simulink model "Demo_1_3Q_ST250"  (Simulink 7.7)
settings: Solver=ode4  StartTime=0.0  StopTime=inf  FixedStep=sample_time_Vicon  RelTol=1e-3
InitFcn:
  | sample_time_Vicon = 0.004;
  | sample_time=0.02;
  | DeltaT = sample_time;
  | H0 = -0.36;
  | Kl = 1;
  | Omega_r =1.1; %1.3
undefined symbols (not defined in the file or in its folder): DiscIntNeverNeededParam
libraries: simulink x19, dspadpt3 x8
(part 1 of 3)
settings Model: Creator=ttcl3  LastModifiedBy=Vicon
settings SolverCC: MaxConsecutiveMinStep=auto
settings DebuggingCC: MultiTaskRateTransMsg=warning
settings SFSimCC: SimParseCustomCode=off

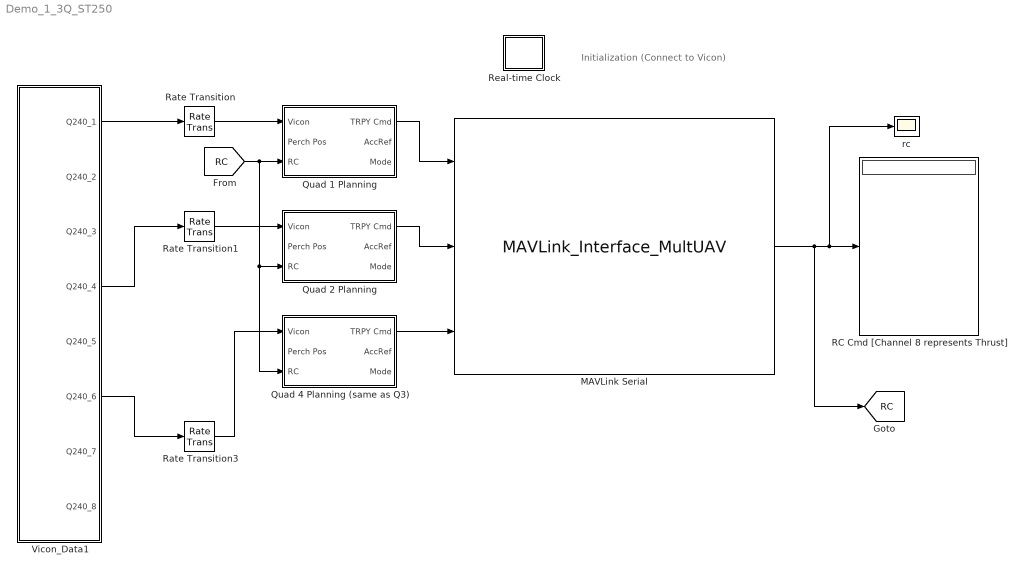
== system Demo_1_3Q_ST250 ==
  note: Initialization
      | (Connect to Vicon)
  MAVLink Serial : S-Function  FunctionName=MAVLink_Interface_MultUAV  Parameters=COM_Port,Baud_Rate,MSG_INPUT,MSG_OUTPUT  EnableBusSupport=off  mask{COM_Port='COM4', Baud_Rate=57600, RC_SCALED=on, Quad_1=on, Quad_2=on, Quad_3=on}
      mask prompts: COM_Port "COM Port"; Baud_Rate "Baud Rate"; RC_SCALED "RC CHANNELS SCALED"; Quad_1 "Quad No 1"; Quad_2 "Quad No 2"; Quad_3 "Quad No 3"
      mask init:
      | MSG_ID_NUM_INPUT = [uint8(196) uint8(197) uint8(198)];
      | MSG_ID_NAME_INPUT = [Quad_1 Quad_2 Quad_3];
      | 
      | MSG_ID_NUM_OUTPUT = [uint8(34)];
      | MSG_ID_NAME_OUTPUT = [RC_SCALED];
      | 
      | idx_input = find(MSG_ID_NAME_INPUT);
      | MSG_INPUT = MSG_ID_NUM_INPUT(idx_input);
      | 
      | idx_output = find(MSG_ID_NAME_OUTPUT);
      | MSG_OUTPUT = MSG_ID_NUM_OUTPUT(idx_output);
      mask TabNameString: Setting,Setting,Output Message,Input Message,Input Message,Input Message
      mask Display:
      | % Block image
      | image(imread('10-inch Quad Heat Map.png'));
      | 
      | %Label block
      | fprintf('MAVLink Serial\n%s\n%dbps', COM_Port,  Baud_Rate)
      | 
      | 
      | %Label input ports
      | 
      | in = 1;
      | if (Quad_1 == 1)
      |     port_label('input', in, 'Quad 1');
      |     in = in + 1;
      | end
      | if (Quad_2 == 1)
      |     port_label('input', in, 'Quad 2');
      |     in = in + 1;
      | end
      | 
      | if (Quad_3 == 1)
      |     port_label('input', in, 'Quad 3');
      |     in = in + 1;
      | end
      | 
      | %Label output ports
      | 
      | out = 1;
      | if (RC_SCALED == 1)
      |     port_label('output', out, 'RC CMD');
      |     out = out + 1;
      | end
  Quad 1 Planning : Subsystem
  Quad 2 Planning : Subsystem
  Quad 4 Planning (same as Q3) : Subsystem
  RC Cmd [Channel 8 represents Thrust] : Display
  Rate Transition : RateTransition  OutPortSampleTime=0.02
  Rate Transition1 : RateTransition  OutPortSampleTime=0.02
  Rate Transition3 : RateTransition  OutPortSampleTime=0.02
  Real-time Clock : Subsystem  mask(Real-time Clock){sample_time=sample_time, tolerance=1}
      mask prompts: sample_time "Synchronize with real-time every n seconds:"; tolerance "Real-time warning tolerance (seconds):"
      mask help: Real-time Synchronization Block
      mask Help: This block synchronizes simulation time with the PC real-time clock or UNIX system clock. The first dialog entry is the period at which the clock is checked to insure real-time synchronization. The second dialog entry is the number of seconds that the simulation time must be within real-time before a warning is printed.
      mask Display: plot(0,0,100,100,[40,60,60,54,54,64,69,76,82,77,81,83,83,81,78,74,70,64,57,49,41,35,32,30,30,31,34,40,47,47,40,40],[90,90,85,85,80,79,76,87,80,70,64,57,49,41,33,28,24,22,21,23,25,31,37,46,56,65,73,78,80,85,85,90],[69,53,53],[64,50,73])
  Vicon_Data1 : Subsystem
  rc : Scope
      settings: TimeRange=10  YMin=-1  YMax=0.1
  tag scope: RC=global
  wires:
  [RC] -> Quad 1 Planning/3(RC), Quad 2 Planning/3(RC), Quad 4 Planning (same as Q3)/3(RC)
  Quad 1 Planning/1(TRPY Cmd) -> MAVLink Serial/1
  Quad 2 Planning/1(TRPY Cmd) -> MAVLink Serial/2
  MAVLink Serial/1 -> [RC], RC Cmd [Channel 8 represents Thrust]/1, rc/1
  Rate Transition/1 -> Quad 1 Planning/1(Vicon)
  Rate Transition1/1 -> Quad 2 Planning/1(Vicon)
  Rate Transition3/1 -> Quad 4 Planning (same as Q3)/1(Vicon)
  Quad 4 Planning (same as Q3)/1(TRPY Cmd) -> MAVLink Serial/3
  Vicon_Data1/1(Q240_1) -> Rate Transition/1
  Vicon_Data1/4(Q240_4) -> Rate Transition1/1
  Vicon_Data1/6(Q240_6) -> Rate Transition3/1

== system Demo_1_3Q_ST250/Quad 1 Planning ==
  Vicon : Inport
  Perch Pos : Inport  Port=2
  RC : Inport  Port=3
  Bus Creator : BusCreator  Inputs=8
  Bus Selector : BusSelector  OutputSignals=Position,Attitude,Velocity,Acceleration
  Horizontal Pos controller : Subsystem
  Mixer : Subsystem
  Rate Transition : RateTransition  OutPortSampleTime=sample_time
  Rate Transition1 : RateTransition  OutPortSampleTime=sample_time
  Trajectory Logic : Subsystem
  Vertical Controller : Subsystem
  Yaw Controller : Subsystem
  TRPY Cmd : Outport
  AccRef : Outport  Port=2
  Mode : Outport  Port=3
  wires:
  Horizontal Pos controller/1(RPY) -> Mixer/1(RP)
  Rate Transition/1 -> Bus Creator/3  "velocity"
  Rate Transition1/1 -> Bus Creator/7  "rc"
  Bus Creator/1 -> Horizontal Pos controller/1(UAV Bus), Yaw Controller/1(UAV Bus), Vertical Controller/1(UAV bus), Trajectory Logic/1(UAV Bus)  "UAV Bus"
  Yaw Controller/1(Yaw rate des) -> Mixer/3(Yaw rate)
  Vertical Controller/1(T) -> Mixer/2(T)
  Bus Selector/4 -> Bus Creator/8  "<Acceleration>"
  Trajectory Logic/1(PosRef) -> Bus Creator/4  "position des"
  Trajectory Logic/2(attitude des) -> Bus Creator/5  "attitude des"
  Trajectory Logic/3(VelRef) -> Bus Creator/6  "velocity des"
  Trajectory Logic/5(HoverThrottle) -> Vertical Controller/2(Hover Throttle)  "Hover Throttle"
  Bus Selector/1 -> Bus Creator/1  "<Position>"
  Bus Selector/2 -> Bus Creator/2  "<Attitude>"
  Bus Selector/3 -> Rate Transition/1  "<Velocity>"
  Vicon/1 -> Bus Selector/1
  Mixer/1(XYZ RPY) -> TRPY Cmd/1
  Trajectory Logic/4(AccRef) -> AccRef/1
  Perch Pos/1 -> Trajectory Logic/2(PerchPos)
  Trajectory Logic/6(Mode) -> Mode/1
  RC/1 -> Rate Transition1/1

== system Demo_1_3Q_ST250/Quad 2 Planning ==
  Vicon : Inport
  Perch Pos : Inport  Port=2
  RC : Inport  Port=3
  Bus Creator : BusCreator  Inputs=8
  Bus Selector : BusSelector  OutputSignals=Position,Attitude,Velocity,Acceleration
  Horizontal Pos controller : Subsystem
  Mixer : Subsystem
  Rate Transition : RateTransition  OutPortSampleTime=sample_time
  Rate Transition1 : RateTransition  OutPortSampleTime=sample_time
  Trajectory Logic : Subsystem
  Vertical Controller : Subsystem
  Yaw Controller : Subsystem
  TRPY Cmd : Outport
  AccRef : Outport  Port=2
  Mode : Outport  Port=3
  wires:
  RC/1 -> Rate Transition1/1
  Trajectory Logic/6(Mode) -> Mode/1
  Perch Pos/1 -> Trajectory Logic/2(PerchPos)
  Trajectory Logic/4(AccRef) -> AccRef/1
  Mixer/1(XYZ RPY) -> TRPY Cmd/1
  Vicon/1 -> Bus Selector/1
  Bus Selector/3 -> Rate Transition/1  "<Velocity>"
  Bus Selector/2 -> Bus Creator/2  "<Attitude>"
  Bus Selector/1 -> Bus Creator/1  "<Position>"
  Trajectory Logic/5(HoverThrottle) -> Vertical Controller/2(Hover Throttle)  "Hover Throttle"
  Trajectory Logic/3(VelRef) -> Bus Creator/6  "velocity des"
  Trajectory Logic/2(attitude des) -> Bus Creator/5  "attitude des"
  Trajectory Logic/1(PosRef) -> Bus Creator/4  "position des"
  Bus Selector/4 -> Bus Creator/8  "<Acceleration>"
  Vertical Controller/1(T) -> Mixer/2(T)
  Yaw Controller/1(Yaw rate des) -> Mixer/3(Yaw rate)
  Bus Creator/1 -> Trajectory Logic/1(UAV Bus), Vertical Controller/1(UAV bus), Yaw Controller/1(UAV Bus), Horizontal Pos controller/1(UAV Bus)  "UAV Bus"
  Rate Transition1/1 -> Bus Creator/7  "rc"
  Rate Transition/1 -> Bus Creator/3  "velocity"
  Horizontal Pos controller/1(RPY) -> Mixer/1(RP)

== system Demo_1_3Q_ST250/Quad 4 Planning (same as Q3) ==
  Vicon : Inport
  Perch Pos : Inport  Port=2
  RC : Inport  Port=3
  Bus Creator : BusCreator  Inputs=8
  Bus Selector : BusSelector  OutputSignals=Position,Attitude,Velocity,Acceleration
  Horizontal Pos controller : Subsystem
  Mixer : Subsystem
  Rate Transition : RateTransition  OutPortSampleTime=sample_time
  Rate Transition1 : RateTransition  OutPortSampleTime=sample_time
  Trajectory Logic : Subsystem
  Vertical Controller : Subsystem
  Yaw Controller : Subsystem
  TRPY Cmd : Outport
  AccRef : Outport  Port=2
  Mode : Outport  Port=3
  wires:
  Horizontal Pos controller/1(RPY) -> Mixer/1(RP)
  Rate Transition/1 -> Bus Creator/3  "velocity"
  Rate Transition1/1 -> Bus Creator/7  "rc"
  Bus Creator/1 -> Horizontal Pos controller/1(UAV Bus), Yaw Controller/1(UAV Bus), Vertical Controller/1(UAV bus), Trajectory Logic/1(UAV Bus)  "UAV Bus"
  Yaw Controller/1(Yaw rate des) -> Mixer/3(Yaw rate)
  Vertical Controller/1(T) -> Mixer/2(T)
  Bus Selector/4 -> Bus Creator/8  "<Acceleration>"
  Trajectory Logic/1(PosRef) -> Bus Creator/4  "position des"
  Trajectory Logic/2(attitude des) -> Bus Creator/5  "attitude des"
  Trajectory Logic/3(VelRef) -> Bus Creator/6  "velocity des"
  Trajectory Logic/5(HoverThrottle) -> Vertical Controller/2(Hover Throttle)  "Hover Throttle"
  Bus Selector/1 -> Bus Creator/1  "<Position>"
  Bus Selector/2 -> Bus Creator/2  "<Attitude>"
  Bus Selector/3 -> Rate Transition/1  "<Velocity>"
  Vicon/1 -> Bus Selector/1
  Mixer/1(XYZ RPY) -> TRPY Cmd/1
  Trajectory Logic/4(AccRef) -> AccRef/1
  Perch Pos/1 -> Trajectory Logic/2(PerchPos)
  Trajectory Logic/6(Mode) -> Mode/1
  RC/1 -> Rate Transition1/1

== system Demo_1_3Q_ST250/Real-time Clock ==
  Real-time Clock : S-Function  FunctionName=rtclock  Parameters=sample_time, tolerance  EnableBusSupport=off

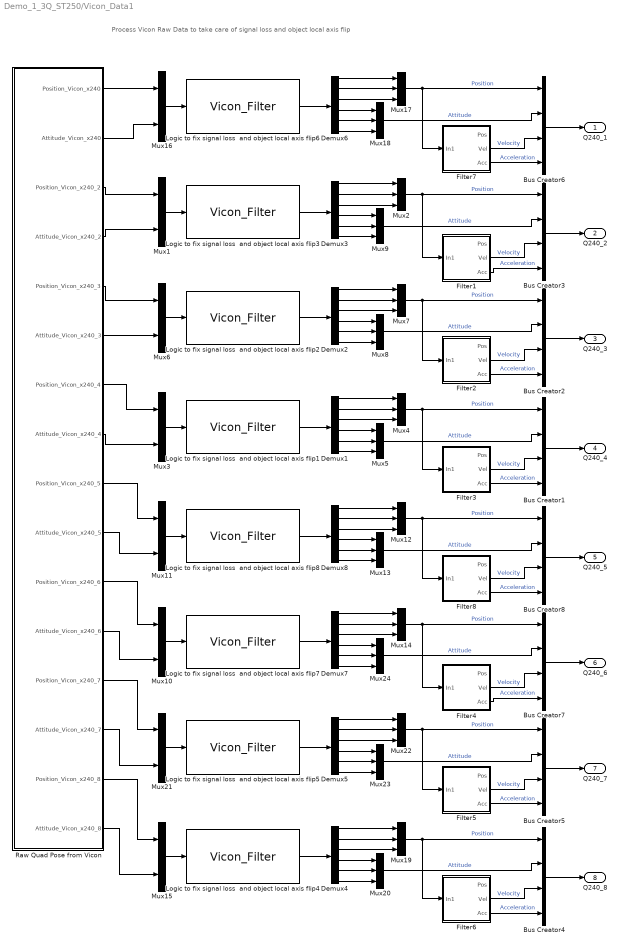
== system Demo_1_3Q_ST250/Vicon_Data1 ==
  note: Process Vicon Raw Data to take care of signal loss and object local axis flip
  Bus Creator{1..8} (8 alike) : BusCreator
  Demux{1..8} (8 alike) : Demux  Outputs=6
  Filter1 : Subsystem
  Filter2 : Subsystem
  Filter3 : Subsystem
  Filter4 : Subsystem
  Filter5 : Subsystem
  Filter6 : Subsystem
  Filter7 : Subsystem
  Filter8 : Subsystem
  Logic to fix signal loss  and object local axis flip{1..8} (8 alike) : M-S-Function  FunctionName=Vicon_Filter
  Mux{1,3,6,10..11,15..16,21} (8 alike) : Mux  Inputs=2
  Mux{2,4..5,7..9,12..14,17..20,22..24} (16 alike) : Mux  Inputs=3
  Raw Quad Pose from Vicon : Subsystem
  Q240_1 : Outport
  Q240_2 : Outport  Port=2
  Q240_3 : Outport  Port=3
  Q240_4 : Outport  Port=4
  Q240_5 : Outport  Port=5
  Q240_6 : Outport  Port=6
  Q240_7 : Outport  Port=7
  Q240_8 : Outport  Port=8
  wires:
  Mux6/1 -> Logic to fix signal loss  and object local axis flip2/1
  Logic to fix signal loss  and object local axis flip2/1 -> Demux2/1
  Demux2/1 -> Mux7/1
  Demux2/2 -> Mux7/2
  Demux2/3 -> Mux7/3
  Demux2/4 -> Mux8/1
  Demux2/5 -> Mux8/2
  Demux2/6 -> Mux8/3
  Filter2/2(Vel) -> Bus Creator2/3  "Velocity"
  Mux7/1 -> Bus Creator2/1, Filter2/1(In1)  "Position"
  Filter2/3(Acc) -> Bus Creator2/4  "Acceleration"
  Mux8/1 -> Bus Creator2/2  "Attitude"
  Bus Creator2/1 -> Q240_3/1
  Mux1/1 -> Logic to fix signal loss  and object local axis flip3/1
  Logic to fix signal loss  and object local axis flip3/1 -> Demux3/1
  Demux3/1 -> Mux2/1
  Demux3/2 -> Mux2/2
  Demux3/3 -> Mux2/3
  Demux3/4 -> Mux9/1
  Demux3/5 -> Mux9/2
  Demux3/6 -> Mux9/3
  Filter1/2(Vel) -> Bus Creator3/3  "Velocity"
  Mux2/1 -> Bus Creator3/1, Filter1/1(In1)  "Position"
  Filter1/3(Acc) -> Bus Creator3/4  "Acceleration"
  Mux9/1 -> Bus Creator3/2  "Attitude"
  Bus Creator3/1 -> Q240_2/1
  Mux16/1 -> Logic to fix signal loss  and object local axis flip6/1
  Logic to fix signal loss  and object local axis flip6/1 -> Demux6/1
  Demux6/1 -> Mux17/1
  Demux6/2 -> Mux17/2
  Demux6/3 -> Mux17/3
  Demux6/4 -> Mux18/1
  Demux6/5 -> Mux18/2
  Demux6/6 -> Mux18/3
  Filter7/2(Vel) -> Bus Creator6/3  "Velocity"
  Mux17/1 -> Bus Creator6/1, Filter7/1(In1)  "Position"
  Filter7/3(Acc) -> Bus Creator6/4  "Acceleration"
  Mux18/1 -> Bus Creator6/2  "Attitude"
  Bus Creator6/1 -> Q240_1/1
  Raw Quad Pose from Vicon/1(Position_Vicon_x240) -> Mux16/1
  Raw Quad Pose from Vicon/2(Attitude_Vicon_x240) -> Mux16/2
  Raw Quad Pose from Vicon/3(Position_Vicon_x240_2) -> Mux1/1
  Raw Quad Pose from Vicon/4(Attitude_Vicon_x240_2) -> Mux1/2
  Mux3/1 -> Logic to fix signal loss  and object local axis flip1/1
  Logic to fix signal loss  and object local axis flip1/1 -> Demux1/1
  Demux1/2 -> Mux4/2
  Demux1/3 -> Mux4/3
  Demux1/4 -> Mux5/1
  Demux1/5 -> Mux5/2
  Demux1/6 -> Mux5/3
  Filter3/2(Vel) -> Bus Creator1/3  "Velocity"
  Mux4/1 -> Filter3/1(In1), Bus Creator1/1  "Position"
  Filter3/3(Acc) -> Bus Creator1/4  "Acceleration"
  Mux5/1 -> Bus Creator1/2  "Attitude"
  Bus Creator1/1 -> Q240_4/1
  Demux1/1 -> Mux4/1
  Raw Quad Pose from Vicon/5(Position_Vicon_x240_3) -> Mux6/1
  Raw Quad Pose from Vicon/6(Attitude_Vicon_x240_3) -> Mux6/2
  Raw Quad Pose from Vicon/7(Position_Vicon_x240_4) -> Mux3/1
  Raw Quad Pose from Vicon/8(Attitude_Vicon_x240_4) -> Mux3/2
  Mux21/1 -> Logic to fix signal loss  and object local axis flip5/1
  Logic to fix signal loss  and object local axis flip5/1 -> Demux5/1
  Demux5/1 -> Mux22/1
  Demux5/2 -> Mux22/2
  Demux5/3 -> Mux22/3
  Demux5/4 -> Mux23/1
  Demux5/5 -> Mux23/2
  Demux5/6 -> Mux23/3
  Filter5/2(Vel) -> Bus Creator5/3  "Velocity"
  Mux22/1 -> Filter5/1(In1), Bus Creator5/1  "Position"
  Filter5/3(Acc) -> Bus Creator5/4  "Acceleration"
  Mux23/1 -> Bus Creator5/2  "Attitude"
  Bus Creator5/1 -> Q240_7/1
  Mux10/1 -> Logic to fix signal loss  and object local axis flip7/1
  Logic to fix signal loss  and object local axis flip7/1 -> Demux7/1
  Demux7/1 -> Mux14/1
  Demux7/2 -> Mux14/2
  Demux7/3 -> Mux14/3
  Demux7/4 -> Mux24/1
  Demux7/5 -> Mux24/2
  Demux7/6 -> Mux24/3
  Filter4/2(Vel) -> Bus Creator7/3  "Velocity"
  Mux14/1 -> Filter4/1(In1), Bus Creator7/1  "Position"
  Filter4/3(Acc) -> Bus Creator7/4  "Acceleration"
  Mux24/1 -> Bus Creator7/2  "Attitude"
  Bus Creator7/1 -> Q240_6/1
  Mux11/1 -> Logic to fix signal loss  and object local axis flip8/1
  Logic to fix signal loss  and object local axis flip8/1 -> Demux8/1
  Demux8/1 -> Mux12/1
  Demux8/2 -> Mux12/2
  Demux8/3 -> Mux12/3
  Demux8/4 -> Mux13/1
  Demux8/5 -> Mux13/2
  Demux8/6 -> Mux13/3
  Filter8/2(Vel) -> Bus Creator8/3  "Velocity"
  Mux12/1 -> Filter8/1(In1), Bus Creator8/1  "Position"
  Filter8/3(Acc) -> Bus Creator8/4  "Acceleration"
  Mux13/1 -> Bus Creator8/2  "Attitude"
  Bus Creator8/1 -> Q240_5/1
  Mux15/1 -> Logic to fix signal loss  and object local axis flip4/1
  Logic to fix signal loss  and object local axis flip4/1 -> Demux4/1
  Demux4/2 -> Mux19/2
  Demux4/3 -> Mux19/3
  Demux4/4 -> Mux20/1
  Demux4/5 -> Mux20/2
  Demux4/6 -> Mux20/3
  Filter6/2(Vel) -> Bus Creator4/3  "Velocity"
  Mux19/1 -> Bus Creator4/1, Filter6/1(In1)  "Position"
  Filter6/3(Acc) -> Bus Creator4/4  "Acceleration"
  Mux20/1 -> Bus Creator4/2  "Attitude"
  Bus Creator4/1 -> Q240_8/1
  Demux4/1 -> Mux19/1
  Raw Quad Pose from Vicon/9(Position_Vicon_x240_5) -> Mux11/1
  Raw Quad Pose from Vicon/10(Attitude_Vicon_x240_5) -> Mux11/2
  Raw Quad Pose from Vicon/11(Position_Vicon_x240_6) -> Mux10/1
  Raw Quad Pose from Vicon/12(Attitude_Vicon_x240_6) -> Mux10/2
  Raw Quad Pose from Vicon/13(Position_Vicon_x240_7) -> Mux21/1
  Raw Quad Pose from Vicon/14(Attitude_Vicon_x240_7) -> Mux21/2
  Raw Quad Pose from Vicon/15(Position_Vicon_x240_8) -> Mux15/1
  Raw Quad Pose from Vicon/16(Attitude_Vicon_x240_8) -> Mux15/2

== system Demo_1_3Q_ST250/Quad 1 Planning/Horizontal Pos controller ==
  UAV Bus : Inport
  Bus Selector : BusSelector  OutputSignals=Position,Attitude,velocity,position des,attitude des,velocity des,rc
  Horizontal Position Controller : Subsystem
  Mux1 : Mux  Inputs=2
  Mux2 : Mux  Inputs=2
  "P Ref1 " : Scope
      settings: TimeRange=10  YMin=-1.5  YMax=1.5  SaveName=ScopeData2
  Pd VS P (Q1) : Scope
      settings: TimeRange=10  YMin=-0.5  YMax=1.5  SaveName=ScopeData16
  Vd VS V : Scope
      settings: TimeRange=10  YMin=-4  YMax=4
  RPY : Outport
  wires:
  UAV Bus/1 -> Horizontal Position Controller/1(UAV Bus), Bus Selector/1
  Horizontal Position Controller/1(RPY) -> RPY/1
  Bus Selector/2 -> ?  "<Attitude>"
  Bus Selector/3 -> Mux2/1  "<velocity>"
  Bus Selector/5 -> ?  "<attitude des>"
  Bus Selector/1 -> Mux1/1, "P Ref1 "/1  "<Position>"
  Bus Selector/4 -> Mux1/2  "<position des>"
  Mux1/1 -> Pd VS P (Q1)/1
  Bus Selector/6 -> Mux2/2  "<velocity des>"
  Bus Selector/7 -> ?  "<rc>"
  Mux2/1 -> Vd VS V/1

== system Demo_1_3Q_ST250/Quad 1 Planning/Mixer ==
  note: 7x1 vector (usec, XYZRPY)
  RP : Inport
  T : Inport  Port=2
  Yaw rate : Inport  Port=3
  Mux1 : Mux  Inputs=5
  PWM : Constant  Value=0
  id : Constant
  XYZ RPY : Outport
  wires:
  Mux1/1 -> XYZ RPY/1
  T/1 -> Mux1/1
  RP/1 -> Mux1/2
  Yaw rate/1 -> Mux1/3
  PWM/1 -> Mux1/4
  id/1 -> Mux1/5

== system Demo_1_3Q_ST250/Quad 1 Planning/Trajectory Logic ==
  UAV Bus : Inport
  PerchPos : Inport  Port=2
  Bus Selector : BusSelector  OutputSignals=rc,Position,Attitude
  CommandRefSystem : Subsystem
  Mux : Mux  Inputs=2
  Selector1 : Selector  InputPortWidth=3  IndexOptions=Index vector (dialog)  Indices=[3]  OutputSizes=1
  UAV SF : Stateflow chart  TreatAsAtomicUnit=on
  PosRef : Outport
  attitude des : Outport  Port=2
  VelRef : Outport  Port=3
  AccRef : Outport  Port=4
  HoverThrottle : Outport  Port=5
  Mode : Outport  Port=6
  wires:
  UAV SF/1(PosDesired) -> CommandRefSystem/1(PosCom)
  CommandRefSystem/1(position des) -> PosRef/1
  CommandRefSystem/3(velocity des) -> VelRef/1
  Bus Selector/1 -> UAV SF/1(RC)  "<rc>"
  CommandRefSystem/4(acc des) -> AccRef/1
  UAV SF/2(HoverThrottle) -> HoverThrottle/1
  PerchPos/1 -> UAV SF/3(PerchPos)
  UAV SF/3(Mode) -> Mode/1
  UAV Bus/1 -> Bus Selector/1
  CommandRefSystem/2(attitude des) -> attitude des/1
  Bus Selector/2 -> Mux/1  "<Position>"
  Bus Selector/3 -> Selector1/1  "<Attitude>"
  Selector1/1 -> Mux/2
  Mux/1 -> UAV SF/2(Pos)

== system Demo_1_3Q_ST250/Quad 1 Planning/Vertical Controller ==
  note: Manual Thrust
  UAV bus : Inport
  Hover Throttle : Inport  Port=2
  Bus Selector : BusSelector  OutputSignals=Position,position des,rc,velocity,velocity des
  Bus Selector3 : BusSelector  OutputSignals=rc
  Selector{1,3..5} (4 alike) : Selector  InputPortWidth=3  IndexOptions=Index vector (dialog)  Indices=[3]  OutputSizes=1
  Selector2 : Selector  InputPortWidth=8  IndexOptions=Index vector (dialog)  Indices=[1]  OutputSizes=1
  Selector7 : Selector  InputPortWidth=8  IndexOptions=Index vector (dialog)  Indices=[7]  OutputSizes=1
  Sum : Sum  Inputs=|-+
  Sum1 : Sum  Inputs=|-+
  Verticall Pos Controller : Subsystem
  T : Outport
  wires:
  UAV bus/1 -> Bus Selector/1
  Bus Selector/3 -> Bus Selector3/1, Selector2/1  "<rc>"
  Bus Selector/1 -> Selector4/1  "<Position>"
  Bus Selector/2 -> Selector1/1  "<position des>"
  Sum/1 -> Verticall Pos Controller/1(Pos Error)  "Down error"
  Selector4/1 -> Sum/1
  Selector1/1 -> Sum/2
  Bus Selector3/1 -> Selector7/1  "<rc>"
  Selector7/1 -> Verticall Pos Controller/2(Reset)  "reset"
  Sum1/1 -> Verticall Pos Controller/3(Vel Error)  "Vel_error"
  Selector3/1 -> Sum1/1
  Selector5/1 -> Sum1/2
  Bus Selector/4 -> Selector3/1  "<velocity>"
  Bus Selector/5 -> Selector5/1  "<velocity des>"
  Verticall Pos Controller/1("T  Commands [-1, 1]") -> T/1  "T"
  Hover Throttle/1 -> Verticall Pos Controller/4(Hover Throttle)

== system Demo_1_3Q_ST250/Quad 1 Planning/Yaw Controller ==
  UAV Bus : Inport
  Bus Selector1 : BusSelector  OutputSignals=Attitude,attitude des,rc
  Gain : Gain  Gain=180/pi
  Heading : simulink/Continuous/PID Controller  SystemSampleTime=-1  Controller=PI  TimeDomain=Discrete-time  SampleTime=sample_time  IntegratorMethod=Trapezoidal  FilterMethod=Trapezoidal  Form=Parallel  P=2  I=1  D=0  N=100  InitialConditionSource=internal  InitialConditionForIntegrator=0  InitialConditionForFilter=0  ExternalReset=rising  LimitOutput=on  UpperSaturationLimit=300*pi/180  LowerSaturationLimit=-300*pi/180  LinearizeAsGain=off  AntiWindupMode=none  Kb=1  TrackingMode=off  Kt=1  PParamMin=[]  PParamMax=[]  IParamMin=[]  IParamMax=[]  DParamMin=[]  DParamMax=[]  NParamMin=[]  NParamMax=[]  KbParamMin=[]  KbParamMax=[]  KtParamMin=[]  KtParamMax=[]  POutMin=[]  POutMax=[]  IOutMin=[]  IOutMax=[]  DOutMin=[]  DOutMax=[]  NOutMin=[]  NOutMax=[]  KbOutMin=[]  KbOutMax=[]  KtOutMin=[]  KtOutMax=[]  IntegratorOutMin=[]  IntegratorOutMax=[]  FilterOutMin=[]  FilterOutMax=[]  SumOutMin=[]  SumOutMax=[]  SumI1OutMin=[]  SumI1OutMax=[]  SumI2OutMin=[]  SumI2OutMax=[]  SumI3OutMin=[]  SumI3OutMax=[]  SumDOutMin=[]  SumDOutMax=[]  SaturationOutMin=[]  SaturationOutMax=[]  IntegratorContinuousStateAttributes=''  IntegratorStateMustResolveToSignalObject=off  IntegratorRTWStateStorageClass=Auto  FilterContinuousStateAttributes=''  FilterStateMustResolveToSignalObject=off  FilterRTWStateStorageClass=Auto
  MATLAB Function : Stateflow chart  TreatAsAtomicUnit=on
  Selector5 : Selector  InputPortWidth=3  IndexOptions=Index vector (dialog)  Indices=[3]  OutputSizes=1
  Selector6 : Selector  InputPortWidth=3  IndexOptions=Index vector (dialog)  Indices=[3]  OutputSizes=1
  Selector7 : Selector  InputPortWidth=8  IndexOptions=Index vector (dialog)  Indices=[5]  OutputSizes=1
  Sum1 : Sum  Inputs=|-+
  Yaw rate des : Outport
  wires:
  Gain/1 -> Yaw rate des/1
  Selector5/1 -> Sum1/1
  Selector7/1 -> Heading/2  "reset"
  Heading/1 -> Gain/1  "desire yaw rate"
  Bus Selector1/1 -> Selector5/1  "<Attitude>"
  UAV Bus/1 -> Bus Selector1/1
  MATLAB Function/1(y) -> Heading/1
  Sum1/1 -> MATLAB Function/1(u)
  Selector6/1 -> Sum1/2
  Bus Selector1/2 -> Selector6/1  "<attitude des>"
  Bus Selector1/3 -> Selector7/1  "<rc>"

== system Demo_1_3Q_ST250/Quad 2 Planning/Horizontal Pos controller ==
  UAV Bus : Inport
  Bus Selector : BusSelector  OutputSignals=Position,Attitude,velocity,position des,attitude des,velocity des,rc
  Horizontal Position Controller : Subsystem
  Mux1 : Mux  Inputs=2
  Mux2 : Mux  Inputs=2
  Pd VS P (Q2) : Scope
      settings: TimeRange=10  YMin=-1.9  YMax=0  SaveName=ScopeData16
  Vd VS V : Scope
      settings: TimeRange=10  YMin=-4  YMax=4
  RPY : Outport
  wires:
  Mux2/1 -> Vd VS V/1
  Bus Selector/7 -> ?  "<rc>"
  Bus Selector/6 -> Mux2/2  "<velocity des>"
  Mux1/1 -> Pd VS P (Q2)/1
  Bus Selector/4 -> Mux1/2  "<position des>"
  Bus Selector/1 -> Mux1/1  "<Position>"
  Bus Selector/5 -> ?  "<attitude des>"
  Bus Selector/3 -> Mux2/1  "<velocity>"
  Bus Selector/2 -> ?  "<Attitude>"
  Horizontal Position Controller/1(RPY) -> RPY/1
  UAV Bus/1 -> Bus Selector/1, Horizontal Position Controller/1(UAV Bus)

== system Demo_1_3Q_ST250/Quad 2 Planning/Mixer ==
  note: 7x1 vector (usec, XYZRPY)
  RP : Inport
  T : Inport  Port=2
  Yaw rate : Inport  Port=3
  Mux1 : Mux  Inputs=5
  PWM : Constant  Value=0
  id : Constant  Value=4
  XYZ RPY : Outport
  wires:
  id/1 -> Mux1/5
  PWM/1 -> Mux1/4
  Yaw rate/1 -> Mux1/3
  RP/1 -> Mux1/2
  T/1 -> Mux1/1
  Mux1/1 -> XYZ RPY/1

== system Demo_1_3Q_ST250/Quad 2 Planning/Trajectory Logic ==
  UAV Bus : Inport
  PerchPos : Inport  Port=2
  Bus Selector : BusSelector  OutputSignals=rc,Position,Attitude
  CommandRefSystem : Subsystem
  Mux : Mux  Inputs=2
  Selector1 : Selector  InputPortWidth=3  IndexOptions=Index vector (dialog)  Indices=[3]  OutputSizes=1
  UAV SF : Stateflow chart  TreatAsAtomicUnit=on
  PosRef : Outport
  attitude des : Outport  Port=2
  VelRef : Outport  Port=3
  AccRef : Outport  Port=4
  HoverThrottle : Outport  Port=5
  Mode : Outport  Port=6
  wires:
  Mux/1 -> UAV SF/2(Pos)
  Selector1/1 -> Mux/2
  Bus Selector/3 -> Selector1/1  "<Attitude>"
  Bus Selector/2 -> Mux/1  "<Position>"
  CommandRefSystem/2(attitude des) -> attitude des/1
  UAV Bus/1 -> Bus Selector/1
  UAV SF/3(Mode) -> Mode/1
  PerchPos/1 -> UAV SF/3(PerchPos)
  UAV SF/2(HoverThrottle) -> HoverThrottle/1
  CommandRefSystem/4(acc des) -> AccRef/1
  Bus Selector/1 -> UAV SF/1(RC)  "<rc>"
  CommandRefSystem/3(velocity des) -> VelRef/1
  CommandRefSystem/1(position des) -> PosRef/1
  UAV SF/1(PosDesired) -> CommandRefSystem/1(PosCom)

== system Demo_1_3Q_ST250/Quad 2 Planning/Vertical Controller ==
  note: Manual Thrust
  UAV bus : Inport
  Hover Throttle : Inport  Port=2
  Bus Selector : BusSelector  OutputSignals=Position,position des,rc,velocity,velocity des
  Bus Selector3 : BusSelector  OutputSignals=rc
  Selector{1,3..5} (4 alike) : Selector  InputPortWidth=3  IndexOptions=Index vector (dialog)  Indices=[3]  OutputSizes=1
  Selector2 : Selector  InputPortWidth=8  IndexOptions=Index vector (dialog)  Indices=[1]  OutputSizes=1
  Selector7 : Selector  InputPortWidth=8  IndexOptions=Index vector (dialog)  Indices=[7]  OutputSizes=1
  Sum : Sum  Inputs=|-+
  Sum1 : Sum  Inputs=|-+
  Verticall Pos Controller : Subsystem
  T : Outport
  wires:
  Hover Throttle/1 -> Verticall Pos Controller/4(Hover Throttle)
  Verticall Pos Controller/1("T  Commands [-1, 1]") -> T/1  "T"
  Bus Selector/5 -> Selector5/1  "<velocity des>"
  Bus Selector/4 -> Selector3/1  "<velocity>"
  Selector5/1 -> Sum1/2
  Selector3/1 -> Sum1/1
  Sum1/1 -> Verticall Pos Controller/3(Vel Error)  "Vel_error"
  Selector7/1 -> Verticall Pos Controller/2(Reset)  "reset"
  Bus Selector3/1 -> Selector7/1  "<rc>"
  Selector1/1 -> Sum/2
  Selector4/1 -> Sum/1
  Sum/1 -> Verticall Pos Controller/1(Pos Error)  "Down error"
  Bus Selector/2 -> Selector1/1  "<position des>"
  Bus Selector/1 -> Selector4/1  "<Position>"
  Bus Selector/3 -> Selector2/1, Bus Selector3/1  "<rc>"
  UAV bus/1 -> Bus Selector/1

== system Demo_1_3Q_ST250/Quad 2 Planning/Yaw Controller ==
  UAV Bus : Inport
  Bus Selector1 : BusSelector  OutputSignals=Attitude,attitude des,rc
  Gain : Gain  Gain=180/pi
  Heading : simulink/Continuous/PID Controller  SystemSampleTime=-1  Controller=PI  TimeDomain=Discrete-time  SampleTime=sample_time  IntegratorMethod=Trapezoidal  FilterMethod=Trapezoidal  Form=Parallel  P=2  I=1  D=0  N=100  InitialConditionSource=internal  InitialConditionForIntegrator=0  InitialConditionForFilter=0  ExternalReset=rising  LimitOutput=on  UpperSaturationLimit=300*pi/180  LowerSaturationLimit=-300*pi/180  LinearizeAsGain=off  AntiWindupMode=none  Kb=1  TrackingMode=off  Kt=1  PParamMin=[]  PParamMax=[]  IParamMin=[]  IParamMax=[]  DParamMin=[]  DParamMax=[]  NParamMin=[]  NParamMax=[]  KbParamMin=[]  KbParamMax=[]  KtParamMin=[]  KtParamMax=[]  POutMin=[]  POutMax=[]  IOutMin=[]  IOutMax=[]  DOutMin=[]  DOutMax=[]  NOutMin=[]  NOutMax=[]  KbOutMin=[]  KbOutMax=[]  KtOutMin=[]  KtOutMax=[]  IntegratorOutMin=[]  IntegratorOutMax=[]  FilterOutMin=[]  FilterOutMax=[]  SumOutMin=[]  SumOutMax=[]  SumI1OutMin=[]  SumI1OutMax=[]  SumI2OutMin=[]  SumI2OutMax=[]  SumI3OutMin=[]  SumI3OutMax=[]  SumDOutMin=[]  SumDOutMax=[]  SaturationOutMin=[]  SaturationOutMax=[]  IntegratorContinuousStateAttributes=''  IntegratorStateMustResolveToSignalObject=off  IntegratorRTWStateStorageClass=Auto  FilterContinuousStateAttributes=''  FilterStateMustResolveToSignalObject=off  FilterRTWStateStorageClass=Auto
  MATLAB Function : Stateflow chart  TreatAsAtomicUnit=on
  Selector5 : Selector  InputPortWidth=3  IndexOptions=Index vector (dialog)  Indices=[3]  OutputSizes=1
  Selector6 : Selector  InputPortWidth=3  IndexOptions=Index vector (dialog)  Indices=[3]  OutputSizes=1
  Selector7 : Selector  InputPortWidth=8  IndexOptions=Index vector (dialog)  Indices=[5]  OutputSizes=1
  Sum1 : Sum  Inputs=|-+
  Yaw rate des : Outport
  wires:
  Bus Selector1/3 -> Selector7/1  "<rc>"
  Bus Selector1/2 -> Selector6/1  "<attitude des>"
  Selector6/1 -> Sum1/2
  Sum1/1 -> MATLAB Function/1(u)
  MATLAB Function/1(y) -> Heading/1
  UAV Bus/1 -> Bus Selector1/1
  Bus Selector1/1 -> Selector5/1  "<Attitude>"
  Heading/1 -> Gain/1  "desire yaw rate"
  Selector7/1 -> Heading/2  "reset"
  Selector5/1 -> Sum1/1
  Gain/1 -> Yaw rate des/1

== system Demo_1_3Q_ST250/Quad 4 Planning (same as Q3)/Horizontal Pos controller ==
  UAV Bus : Inport
  Bus Selector : BusSelector  OutputSignals=Position,Attitude,velocity,position des,attitude des,velocity des,rc
  Horizontal Position Controller : Subsystem
  Mux1 : Mux  Inputs=2
  Mux2 : Mux  Inputs=2
  Pd VS P (Q3) : Scope
      settings: TimeRange=10  YMin=-2.25  YMax=1.25  SaveName=ScopeData16
  Vd VS V : Scope
      settings: TimeRange=10  YMin=-4  YMax=4
  RPY : Outport
  wires:
  UAV Bus/1 -> Horizontal Position Controller/1(UAV Bus), Bus Selector/1
  Horizontal Position Controller/1(RPY) -> RPY/1
  Bus Selector/2 -> ?  "<Attitude>"
  Bus Selector/3 -> Mux2/1  "<velocity>"
  Bus Selector/5 -> ?  "<attitude des>"
  Bus Selector/1 -> Mux1/1  "<Position>"
  Bus Selector/4 -> Mux1/2  "<position des>"
  Mux1/1 -> Pd VS P (Q3)/1
  Bus Selector/6 -> Mux2/2  "<velocity des>"
  Bus Selector/7 -> ?  "<rc>"
  Mux2/1 -> Vd VS V/1

== system Demo_1_3Q_ST250/Quad 4 Planning (same as Q3)/Mixer ==
  note: 7x1 vector (usec, XYZRPY)
  RP : Inport
  T : Inport  Port=2
  Yaw rate : Inport  Port=3
  Mux1 : Mux  Inputs=5
  PWM : Constant  Value=0
  id : Constant  Value=6
  XYZ RPY : Outport
  wires:
  Mux1/1 -> XYZ RPY/1
  T/1 -> Mux1/1
  RP/1 -> Mux1/2
  Yaw rate/1 -> Mux1/3
  PWM/1 -> Mux1/4
  id/1 -> Mux1/5

== system Demo_1_3Q_ST250/Quad 4 Planning (same as Q3)/Trajectory Logic ==
  UAV Bus : Inport
  PerchPos : Inport  Port=2
  Bus Selector : BusSelector  OutputSignals=rc,Position,Attitude
  CommandRefSystem : Subsystem
  Mux : Mux  Inputs=2
  Selector1 : Selector  InputPortWidth=3  IndexOptions=Index vector (dialog)  Indices=[3]  OutputSizes=1
  UAV SF : Stateflow chart  TreatAsAtomicUnit=on
  PosRef : Outport
  attitude des : Outport  Port=2
  VelRef : Outport  Port=3
  AccRef : Outport  Port=4
  HoverThrottle : Outport  Port=5
  Mode : Outport  Port=6
  wires:
  UAV SF/1(PosDesired) -> CommandRefSystem/1(PosCom)
  CommandRefSystem/1(position des) -> PosRef/1
  CommandRefSystem/3(velocity des) -> VelRef/1
  Bus Selector/1 -> UAV SF/1(RC)  "<rc>"
  CommandRefSystem/4(acc des) -> AccRef/1
  UAV SF/2(HoverThrottle) -> HoverThrottle/1
  PerchPos/1 -> UAV SF/3(PerchPos)
  UAV SF/3(Mode) -> Mode/1
  UAV Bus/1 -> Bus Selector/1
  CommandRefSystem/2(attitude des) -> attitude des/1
  Bus Selector/2 -> Mux/1  "<Position>"
  Bus Selector/3 -> Selector1/1  "<Attitude>"
  Selector1/1 -> Mux/2
  Mux/1 -> UAV SF/2(Pos)

== system Demo_1_3Q_ST250/Quad 4 Planning (same as Q3)/Vertical Controller ==
  note: Manual Thrust
  UAV bus : Inport
  Hover Throttle : Inport  Port=2
  Bus Selector : BusSelector  OutputSignals=Position,position des,rc,velocity,velocity des
  Bus Selector3 : BusSelector  OutputSignals=rc
  Selector{1,3..5} (4 alike) : Selector  InputPortWidth=3  IndexOptions=Index vector (dialog)  Indices=[3]  OutputSizes=1
  Selector2 : Selector  InputPortWidth=8  IndexOptions=Index vector (dialog)  Indices=[1]  OutputSizes=1
  Selector7 : Selector  InputPortWidth=8  IndexOptions=Index vector (dialog)  Indices=[7]  OutputSizes=1
  Sum : Sum  Inputs=|-+
  Sum1 : Sum  Inputs=|-+
  Verticall Pos Controller : Subsystem
  T : Outport
  wires:
  UAV bus/1 -> Bus Selector/1
  Bus Selector/3 -> Bus Selector3/1, Selector2/1  "<rc>"
  Bus Selector/1 -> Selector4/1  "<Position>"
  Bus Selector/2 -> Selector1/1  "<position des>"
  Sum/1 -> Verticall Pos Controller/1(Pos Error)  "Down error"
  Selector4/1 -> Sum/1
  Selector1/1 -> Sum/2
  Bus Selector3/1 -> Selector7/1  "<rc>"
  Selector7/1 -> Verticall Pos Controller/2(Reset)  "reset"
  Sum1/1 -> Verticall Pos Controller/3(Vel Error)  "Vel_error"
  Selector3/1 -> Sum1/1
  Selector5/1 -> Sum1/2
  Bus Selector/4 -> Selector3/1  "<velocity>"
  Bus Selector/5 -> Selector5/1  "<velocity des>"
  Verticall Pos Controller/1("T  Commands [-1, 1]") -> T/1  "T"
  Hover Throttle/1 -> Verticall Pos Controller/4(Hover Throttle)

== system Demo_1_3Q_ST250/Quad 4 Planning (same as Q3)/Yaw Controller ==
  UAV Bus : Inport
  Bus Selector1 : BusSelector  OutputSignals=Attitude,attitude des,rc
  Gain : Gain  Gain=180/pi
  Heading : simulink/Continuous/PID Controller  SystemSampleTime=-1  Controller=PI  TimeDomain=Discrete-time  SampleTime=sample_time  IntegratorMethod=Trapezoidal  FilterMethod=Trapezoidal  Form=Parallel  P=2  I=1  D=0  N=100  InitialConditionSource=internal  InitialConditionForIntegrator=0  InitialConditionForFilter=0  ExternalReset=rising  LimitOutput=on  UpperSaturationLimit=300*pi/180  LowerSaturationLimit=-300*pi/180  LinearizeAsGain=off  AntiWindupMode=none  Kb=1  TrackingMode=off  Kt=1  PParamMin=[]  PParamMax=[]  IParamMin=[]  IParamMax=[]  DParamMin=[]  DParamMax=[]  NParamMin=[]  NParamMax=[]  KbParamMin=[]  KbParamMax=[]  KtParamMin=[]  KtParamMax=[]  POutMin=[]  POutMax=[]  IOutMin=[]  IOutMax=[]  DOutMin=[]  DOutMax=[]  NOutMin=[]  NOutMax=[]  KbOutMin=[]  KbOutMax=[]  KtOutMin=[]  KtOutMax=[]  IntegratorOutMin=[]  IntegratorOutMax=[]  FilterOutMin=[]  FilterOutMax=[]  SumOutMin=[]  SumOutMax=[]  SumI1OutMin=[]  SumI1OutMax=[]  SumI2OutMin=[]  SumI2OutMax=[]  SumI3OutMin=[]  SumI3OutMax=[]  SumDOutMin=[]  SumDOutMax=[]  SaturationOutMin=[]  SaturationOutMax=[]  IntegratorContinuousStateAttributes=''  IntegratorStateMustResolveToSignalObject=off  IntegratorRTWStateStorageClass=Auto  FilterContinuousStateAttributes=''  FilterStateMustResolveToSignalObject=off  FilterRTWStateStorageClass=Auto
  MATLAB Function : Stateflow chart  TreatAsAtomicUnit=on
  Selector5 : Selector  InputPortWidth=3  IndexOptions=Index vector (dialog)  Indices=[3]  OutputSizes=1
  Selector6 : Selector  InputPortWidth=3  IndexOptions=Index vector (dialog)  Indices=[3]  OutputSizes=1
  Selector7 : Selector  InputPortWidth=8  IndexOptions=Index vector (dialog)  Indices=[5]  OutputSizes=1
  Sum1 : Sum  Inputs=|-+
  Yaw rate des : Outport
  wires:
  Gain/1 -> Yaw rate des/1
  Selector5/1 -> Sum1/1
  Selector7/1 -> Heading/2  "reset"
  Heading/1 -> Gain/1  "desire yaw rate"
  Bus Selector1/1 -> Selector5/1  "<Attitude>"
  UAV Bus/1 -> Bus Selector1/1
  MATLAB Function/1(y) -> Heading/1
  Sum1/1 -> MATLAB Function/1(u)
  Selector6/1 -> Sum1/2
  Bus Selector1/2 -> Selector6/1  "<attitude des>"
  Bus Selector1/3 -> Selector7/1  "<rc>"

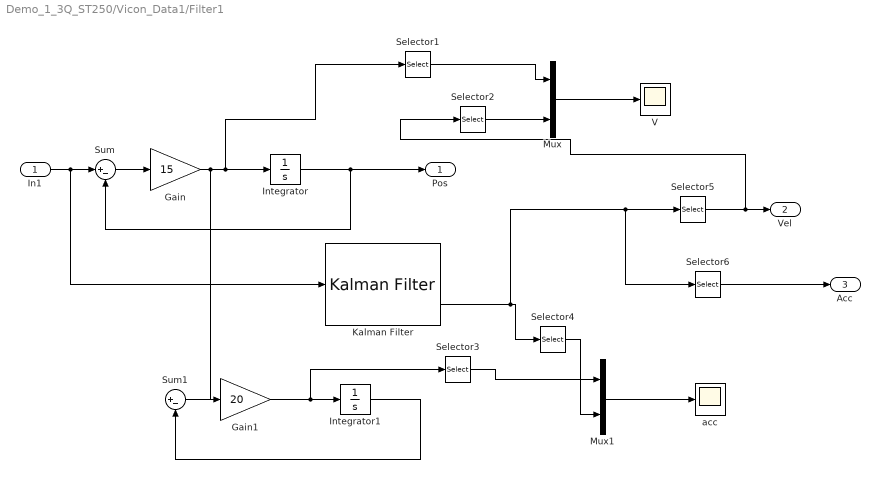
== system Demo_1_3Q_ST250/Vicon_Data1/Filter1 ==
  In1 : Inport
  Gain : Gain  Gain=15
  Gain1 : Gain  Gain=20
  Integrator : Integrator
  Integrator1 : Integrator
  Kalman Filter : dspadpt3/Kalman Filter  SystemSampleTime=-1  num_targets=1  sourceEnable=Always  isReset=on  X=zeros([9, 1])  P=zeros(9)  A=[1 sample_time_Vicon sample_time_Vicon*sample_time_Vicon/2 zeros(1,6);0 1 sample_time_Vicon zeros(1,6);0 0 1 zeros(1,6);0 0 0 1 sample_time_Vicon sample_time_Vicon*sample_time_Vicon/2 0 0 0;zeros(1,4) 1 sample_time_Vicon zeros(1,3);zeros(1,5) 1 zeros(1,3);zeros(1,6) 1 sample_time_Vicon sample_time_Vicon*sample_time_Vicon/2;zeros(1,7) 1 sample_time_Vicon;zeros(1,8) 1]  sourceMeasure=Specify via Dialog  H=[1 zeros(1,8); zeros(1,3) 1 zeros(1,5);zeros(1,6) 1 0 0]  Q=diag([0 0.001 0.001 0 0.001 0.001 0 0.001 0.001])  R=0.001*eye(3)  isOutputEstMeasure=on  isOutputEstState=on  isOutputEstError=off  isOutputPrdMeasure=off  isOutputPrdState=off  isOutputPrdError=off
  Mux : Mux  Inputs=2
  Mux1 : Mux  Inputs=2
  Selector1 : Selector  InputPortWidth=3  IndexOptions=Index vector (dialog)  Indices=[2]  OutputSizes=1
  Selector2 : Selector  InputPortWidth=3  IndexOptions=Index vector (dialog)  Indices=[2]  OutputSizes=1
  Selector3 : Selector  InputPortWidth=3  IndexOptions=Index vector (dialog)  Indices=[2]  OutputSizes=1
  Selector4 : Selector  InputPortWidth=9  IndexOptions=Index vector (dialog)  Indices=[6]  OutputSizes=1
  Selector5 : Selector  InputPortWidth=9  IndexOptions=Index vector (dialog)  Indices=[2 5 8]  OutputSizes=1
  Selector6 : Selector  InputPortWidth=9  IndexOptions=Index vector (dialog)  Indices=[3 6 9]  OutputSizes=1
  Sum : Sum  Inputs=|+-
  Sum1 : Sum  Inputs=|+-
  V : Scope
      settings: YMin=-3.5  YMax=7.5  SaveName=ScopeData3
  acc : Scope
      settings: YMin=-3.5  YMax=7.5  SaveName=ScopeData6
  Pos : Outport
  Vel : Outport  Port=2
  Acc : Outport  Port=3
  wires:
  Selector2/1 -> Mux/2
  Selector1/1 -> Mux/1
  Mux1/1 -> acc/1
  Selector5/1 -> Selector2/1, Vel/1
  Mux/1 -> V/1
  Sum/1 -> Gain/1
  Gain/1 -> Selector1/1, Integrator/1, Sum1/1
  Integrator/1 -> Pos/1, Sum/2
  In1/1 -> Kalman Filter/1, Sum/1
  Kalman Filter/2 -> Selector4/1, Selector5/1, Selector6/1
  Sum1/1 -> Gain1/1
  Gain1/1 -> Integrator1/1, Selector3/1
  Integrator1/1 -> Sum1/2
  Selector3/1 -> Mux1/1
  Selector4/1 -> Mux1/2
  Selector6/1 -> Acc/1

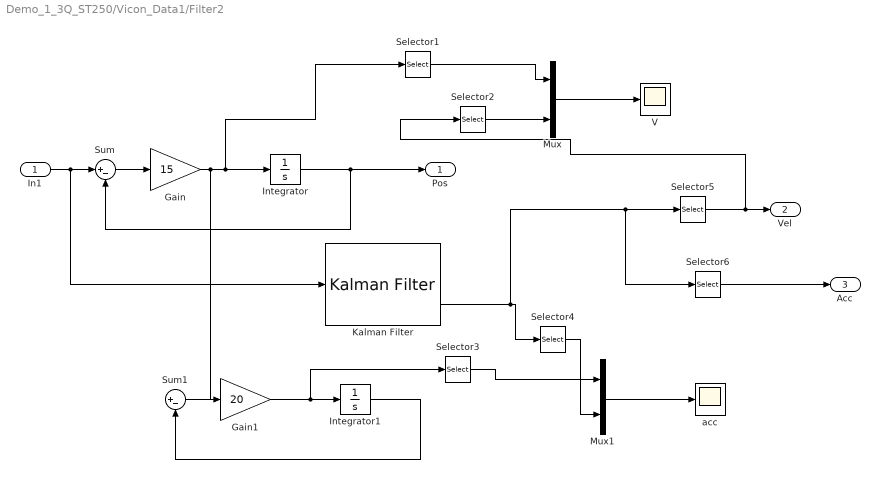
== system Demo_1_3Q_ST250/Vicon_Data1/Filter2 ==
  In1 : Inport
  Gain : Gain  Gain=15
  Gain1 : Gain  Gain=20
  Integrator : Integrator
  Integrator1 : Integrator
  Kalman Filter : dspadpt3/Kalman Filter  SystemSampleTime=-1  num_targets=1  sourceEnable=Always  isReset=on  X=zeros([9, 1])  P=zeros(9)  A=[1 sample_time_Vicon sample_time_Vicon*sample_time_Vicon/2 zeros(1,6);0 1 sample_time_Vicon zeros(1,6);0 0 1 zeros(1,6);0 0 0 1 sample_time_Vicon sample_time_Vicon*sample_time_Vicon/2 0 0 0;zeros(1,4) 1 sample_time_Vicon zeros(1,3);zeros(1,5) 1 zeros(1,3);zeros(1,6) 1 sample_time_Vicon sample_time_Vicon*sample_time_Vicon/2;zeros(1,7) 1 sample_time_Vicon;zeros(1,8) 1]  sourceMeasure=Specify via Dialog  H=[1 zeros(1,8); zeros(1,3) 1 zeros(1,5);zeros(1,6) 1 0 0]  Q=diag([0 0.001 0.001 0 0.001 0.001 0 0.001 0.001])  R=0.001*eye(3)  isOutputEstMeasure=on  isOutputEstState=on  isOutputEstError=off  isOutputPrdMeasure=off  isOutputPrdState=off  isOutputPrdError=off
  Mux : Mux  Inputs=2
  Mux1 : Mux  Inputs=2
  Selector1 : Selector  InputPortWidth=3  IndexOptions=Index vector (dialog)  Indices=[2]  OutputSizes=1
  Selector2 : Selector  InputPortWidth=3  IndexOptions=Index vector (dialog)  Indices=[2]  OutputSizes=1
  Selector3 : Selector  InputPortWidth=3  IndexOptions=Index vector (dialog)  Indices=[2]  OutputSizes=1
  Selector4 : Selector  InputPortWidth=9  IndexOptions=Index vector (dialog)  Indices=[6]  OutputSizes=1
  Selector5 : Selector  InputPortWidth=9  IndexOptions=Index vector (dialog)  Indices=[2 5 8]  OutputSizes=1
  Selector6 : Selector  InputPortWidth=9  IndexOptions=Index vector (dialog)  Indices=[3 6 9]  OutputSizes=1
  Sum : Sum  Inputs=|+-
  Sum1 : Sum  Inputs=|+-
  V : Scope
      settings: YMin=-3.5  YMax=7.5  SaveName=ScopeData3
  acc : Scope
      settings: YMin=-3.5  YMax=7.5  SaveName=ScopeData6
  Pos : Outport
  Vel : Outport  Port=2
  Acc : Outport  Port=3
  wires:
  Selector6/1 -> Acc/1
  Selector4/1 -> Mux1/2
  Selector3/1 -> Mux1/1
  Integrator1/1 -> Sum1/2
  Gain1/1 -> Selector3/1, Integrator1/1
  Sum1/1 -> Gain1/1
  Kalman Filter/2 -> Selector6/1, Selector5/1, Selector4/1
  In1/1 -> Sum/1, Kalman Filter/1
  Integrator/1 -> Sum/2, Pos/1
  Gain/1 -> Sum1/1, Integrator/1, Selector1/1
  Sum/1 -> Gain/1
  Mux/1 -> V/1
  Selector5/1 -> Vel/1, Selector2/1
  Mux1/1 -> acc/1
  Selector1/1 -> Mux/1
  Selector2/1 -> Mux/2

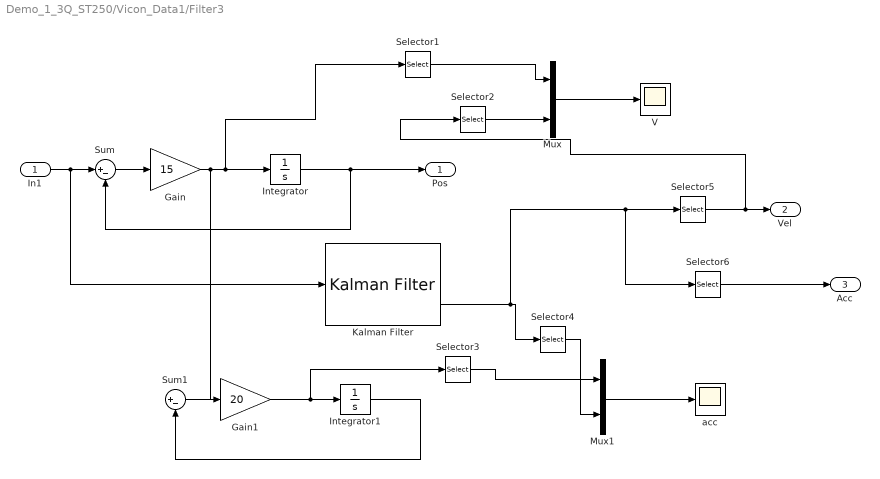
== system Demo_1_3Q_ST250/Vicon_Data1/Filter3 ==
  In1 : Inport
  Gain : Gain  Gain=15
  Gain1 : Gain  Gain=20
  Integrator : Integrator
  Integrator1 : Integrator
  Kalman Filter : dspadpt3/Kalman Filter  SystemSampleTime=-1  num_targets=1  sourceEnable=Always  isReset=on  X=zeros([9, 1])  P=zeros(9)  A=[1 sample_time_Vicon sample_time_Vicon*sample_time_Vicon/2 zeros(1,6);0 1 sample_time_Vicon zeros(1,6);0 0 1 zeros(1,6);0 0 0 1 sample_time_Vicon sample_time_Vicon*sample_time_Vicon/2 0 0 0;zeros(1,4) 1 sample_time_Vicon zeros(1,3);zeros(1,5) 1 zeros(1,3);zeros(1,6) 1 sample_time_Vicon sample_time_Vicon*sample_time_Vicon/2;zeros(1,7) 1 sample_time_Vicon;zeros(1,8) 1]  sourceMeasure=Specify via Dialog  H=[1 zeros(1,8); zeros(1,3) 1 zeros(1,5);zeros(1,6) 1 0 0]  Q=diag([0 0.001 0.001 0 0.001 0.001 0 0.001 0.001])  R=0.001*eye(3)  isOutputEstMeasure=on  isOutputEstState=on  isOutputEstError=off  isOutputPrdMeasure=off  isOutputPrdState=off  isOutputPrdError=off
  Mux : Mux  Inputs=2
  Mux1 : Mux  Inputs=2
  Selector1 : Selector  InputPortWidth=3  IndexOptions=Index vector (dialog)  Indices=[2]  OutputSizes=1
  Selector2 : Selector  InputPortWidth=3  IndexOptions=Index vector (dialog)  Indices=[2]  OutputSizes=1
  Selector3 : Selector  InputPortWidth=3  IndexOptions=Index vector (dialog)  Indices=[2]  OutputSizes=1
  Selector4 : Selector  InputPortWidth=9  IndexOptions=Index vector (dialog)  Indices=[6]  OutputSizes=1
  Selector5 : Selector  InputPortWidth=9  IndexOptions=Index vector (dialog)  Indices=[2 5 8]  OutputSizes=1
  Selector6 : Selector  InputPortWidth=9  IndexOptions=Index vector (dialog)  Indices=[3 6 9]  OutputSizes=1
  Sum : Sum  Inputs=|+-
  Sum1 : Sum  Inputs=|+-
  V : Scope
      settings: YMin=-3.5  YMax=7.5  SaveName=ScopeData3
  acc : Scope
      settings: YMin=-3.5  YMax=7.5  SaveName=ScopeData6
  Pos : Outport
  Vel : Outport  Port=2
  Acc : Outport  Port=3
  wires:
  Selector2/1 -> Mux/2
  Selector1/1 -> Mux/1
  Mux1/1 -> acc/1
  Selector5/1 -> Selector2/1, Vel/1
  Mux/1 -> V/1
  Sum/1 -> Gain/1
  Gain/1 -> Selector1/1, Integrator/1, Sum1/1
  Integrator/1 -> Pos/1, Sum/2
  In1/1 -> Kalman Filter/1, Sum/1
  Kalman Filter/2 -> Selector4/1, Selector5/1, Selector6/1
  Sum1/1 -> Gain1/1
  Gain1/1 -> Integrator1/1, Selector3/1
  Integrator1/1 -> Sum1/2
  Selector3/1 -> Mux1/1
  Selector4/1 -> Mux1/2
  Selector6/1 -> Acc/1

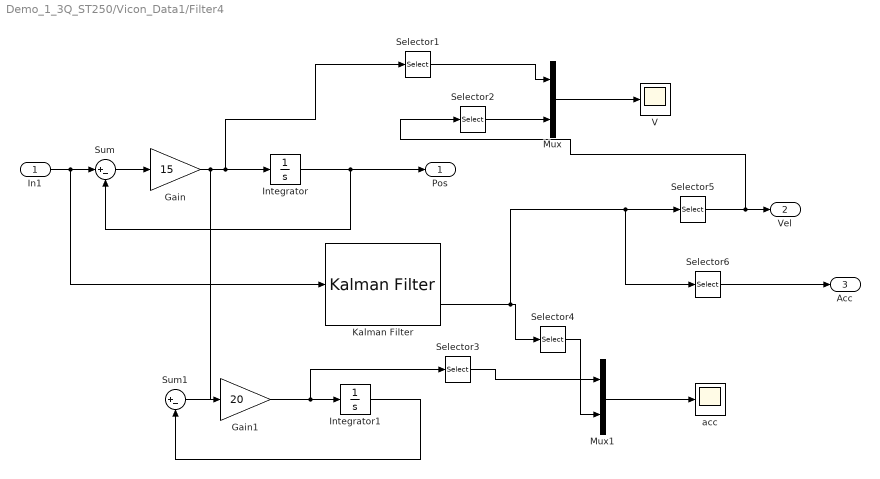
== system Demo_1_3Q_ST250/Vicon_Data1/Filter4 ==
  In1 : Inport
  Gain : Gain  Gain=15
  Gain1 : Gain  Gain=20
  Integrator : Integrator
  Integrator1 : Integrator
  Kalman Filter : dspadpt3/Kalman Filter  SystemSampleTime=-1  num_targets=1  sourceEnable=Always  isReset=on  X=zeros([9, 1])  P=zeros(9)  A=[1 sample_time_Vicon sample_time_Vicon*sample_time_Vicon/2 zeros(1,6);0 1 sample_time_Vicon zeros(1,6);0 0 1 zeros(1,6);0 0 0 1 sample_time_Vicon sample_time_Vicon*sample_time_Vicon/2 0 0 0;zeros(1,4) 1 sample_time_Vicon zeros(1,3);zeros(1,5) 1 zeros(1,3);zeros(1,6) 1 sample_time_Vicon sample_time_Vicon*sample_time_Vicon/2;zeros(1,7) 1 sample_time_Vicon;zeros(1,8) 1]  sourceMeasure=Specify via Dialog  H=[1 zeros(1,8); zeros(1,3) 1 zeros(1,5);zeros(1,6) 1 0 0]  Q=diag([0 0.001 0.001 0 0.001 0.001 0 0.001 0.001])  R=0.001*eye(3)  isOutputEstMeasure=on  isOutputEstState=on  isOutputEstError=off  isOutputPrdMeasure=off  isOutputPrdState=off  isOutputPrdError=off
  Mux : Mux  Inputs=2
  Mux1 : Mux  Inputs=2
  Selector1 : Selector  InputPortWidth=3  IndexOptions=Index vector (dialog)  Indices=[2]  OutputSizes=1
  Selector2 : Selector  InputPortWidth=3  IndexOptions=Index vector (dialog)  Indices=[2]  OutputSizes=1
  Selector3 : Selector  InputPortWidth=3  IndexOptions=Index vector (dialog)  Indices=[2]  OutputSizes=1
  Selector4 : Selector  InputPortWidth=9  IndexOptions=Index vector (dialog)  Indices=[6]  OutputSizes=1
  Selector5 : Selector  InputPortWidth=9  IndexOptions=Index vector (dialog)  Indices=[2 5 8]  OutputSizes=1
  Selector6 : Selector  InputPortWidth=9  IndexOptions=Index vector (dialog)  Indices=[3 6 9]  OutputSizes=1
  Sum : Sum  Inputs=|+-
  Sum1 : Sum  Inputs=|+-
  V : Scope
      settings: YMin=-3.5  YMax=7.5  SaveName=ScopeData3
  acc : Scope
      settings: YMin=-3.5  YMax=7.5  SaveName=ScopeData6
  Pos : Outport
  Vel : Outport  Port=2
  Acc : Outport  Port=3
  wires:
  Selector6/1 -> Acc/1
  Selector4/1 -> Mux1/2
  Selector3/1 -> Mux1/1
  Integrator1/1 -> Sum1/2
  Gain1/1 -> Selector3/1, Integrator1/1
  Sum1/1 -> Gain1/1
  Kalman Filter/2 -> Selector6/1, Selector5/1, Selector4/1
  In1/1 -> Sum/1, Kalman Filter/1
  Integrator/1 -> Sum/2, Pos/1
  Gain/1 -> Sum1/1, Integrator/1, Selector1/1
  Sum/1 -> Gain/1
  Mux/1 -> V/1
  Selector5/1 -> Vel/1, Selector2/1
  Mux1/1 -> acc/1
  Selector1/1 -> Mux/1
  Selector2/1 -> Mux/2

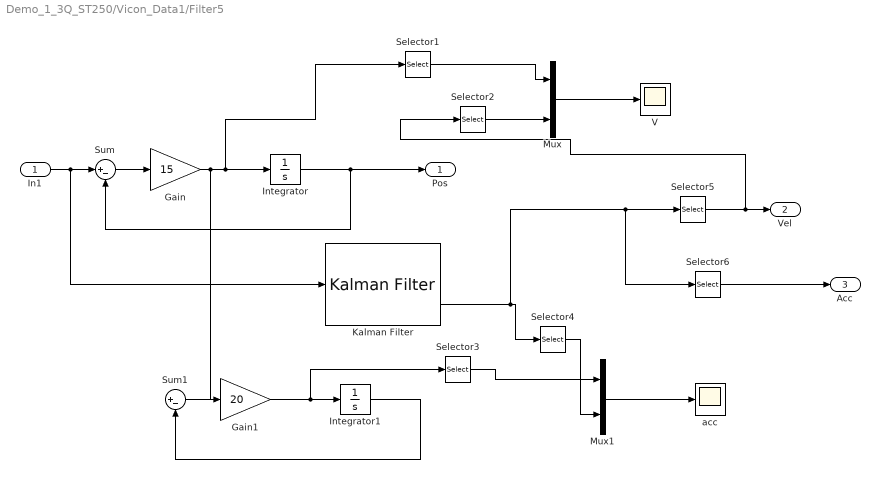
== system Demo_1_3Q_ST250/Vicon_Data1/Filter5 ==
  In1 : Inport
  Gain : Gain  Gain=15
  Gain1 : Gain  Gain=20
  Integrator : Integrator
  Integrator1 : Integrator
  Kalman Filter : dspadpt3/Kalman Filter  SystemSampleTime=-1  num_targets=1  sourceEnable=Always  isReset=on  X=zeros([9, 1])  P=zeros(9)  A=[1 sample_time_Vicon sample_time_Vicon*sample_time_Vicon/2 zeros(1,6);0 1 sample_time_Vicon zeros(1,6);0 0 1 zeros(1,6);0 0 0 1 sample_time_Vicon sample_time_Vicon*sample_time_Vicon/2 0 0 0;zeros(1,4) 1 sample_time_Vicon zeros(1,3);zeros(1,5) 1 zeros(1,3);zeros(1,6) 1 sample_time_Vicon sample_time_Vicon*sample_time_Vicon/2;zeros(1,7) 1 sample_time_Vicon;zeros(1,8) 1]  sourceMeasure=Specify via Dialog  H=[1 zeros(1,8); zeros(1,3) 1 zeros(1,5);zeros(1,6) 1 0 0]  Q=diag([0 0.001 0.001 0 0.001 0.001 0 0.001 0.001])  R=0.001*eye(3)  isOutputEstMeasure=on  isOutputEstState=on  isOutputEstError=off  isOutputPrdMeasure=off  isOutputPrdState=off  isOutputPrdError=off
  Mux : Mux  Inputs=2
  Mux1 : Mux  Inputs=2
  Selector1 : Selector  InputPortWidth=3  IndexOptions=Index vector (dialog)  Indices=[2]  OutputSizes=1
  Selector2 : Selector  InputPortWidth=3  IndexOptions=Index vector (dialog)  Indices=[2]  OutputSizes=1
  Selector3 : Selector  InputPortWidth=3  IndexOptions=Index vector (dialog)  Indices=[2]  OutputSizes=1
  Selector4 : Selector  InputPortWidth=9  IndexOptions=Index vector (dialog)  Indices=[6]  OutputSizes=1
  Selector5 : Selector  InputPortWidth=9  IndexOptions=Index vector (dialog)  Indices=[2 5 8]  OutputSizes=1
  Selector6 : Selector  InputPortWidth=9  IndexOptions=Index vector (dialog)  Indices=[3 6 9]  OutputSizes=1
  Sum : Sum  Inputs=|+-
  Sum1 : Sum  Inputs=|+-
  V : Scope
      settings: YMin=-3.5  YMax=7.5  SaveName=ScopeData3
  acc : Scope
      settings: YMin=-3.5  YMax=7.5  SaveName=ScopeData6
  Pos : Outport
  Vel : Outport  Port=2
  Acc : Outport  Port=3
  wires:
  Selector2/1 -> Mux/2
  Selector1/1 -> Mux/1
  Mux1/1 -> acc/1
  Selector5/1 -> Selector2/1, Vel/1
  Mux/1 -> V/1
  Sum/1 -> Gain/1
  Gain/1 -> Selector1/1, Integrator/1, Sum1/1
  Integrator/1 -> Pos/1, Sum/2
  In1/1 -> Kalman Filter/1, Sum/1
  Kalman Filter/2 -> Selector4/1, Selector5/1, Selector6/1
  Sum1/1 -> Gain1/1
  Gain1/1 -> Integrator1/1, Selector3/1
  Integrator1/1 -> Sum1/2
  Selector3/1 -> Mux1/1
  Selector4/1 -> Mux1/2
  Selector6/1 -> Acc/1

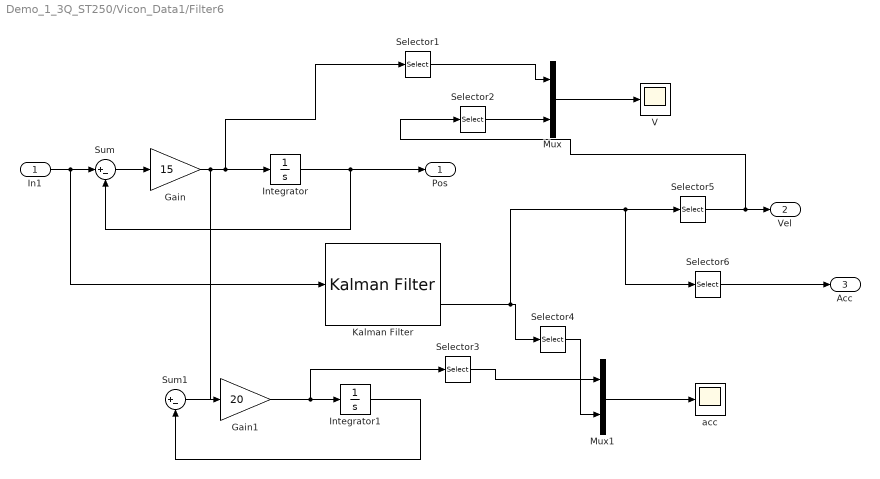
== system Demo_1_3Q_ST250/Vicon_Data1/Filter6 ==
  In1 : Inport
  Gain : Gain  Gain=15
  Gain1 : Gain  Gain=20
  Integrator : Integrator
  Integrator1 : Integrator
  Kalman Filter : dspadpt3/Kalman Filter  SystemSampleTime=-1  num_targets=1  sourceEnable=Always  isReset=on  X=zeros([9, 1])  P=zeros(9)  A=[1 sample_time_Vicon sample_time_Vicon*sample_time_Vicon/2 zeros(1,6);0 1 sample_time_Vicon zeros(1,6);0 0 1 zeros(1,6);0 0 0 1 sample_time_Vicon sample_time_Vicon*sample_time_Vicon/2 0 0 0;zeros(1,4) 1 sample_time_Vicon zeros(1,3);zeros(1,5) 1 zeros(1,3);zeros(1,6) 1 sample_time_Vicon sample_time_Vicon*sample_time_Vicon/2;zeros(1,7) 1 sample_time_Vicon;zeros(1,8) 1]  sourceMeasure=Specify via Dialog  H=[1 zeros(1,8); zeros(1,3) 1 zeros(1,5);zeros(1,6) 1 0 0]  Q=diag([0 0.001 0.001 0 0.001 0.001 0 0.001 0.001])  R=0.001*eye(3)  isOutputEstMeasure=on  isOutputEstState=on  isOutputEstError=off  isOutputPrdMeasure=off  isOutputPrdState=off  isOutputPrdError=off
  Mux : Mux  Inputs=2
  Mux1 : Mux  Inputs=2
  Selector1 : Selector  InputPortWidth=3  IndexOptions=Index vector (dialog)  Indices=[2]  OutputSizes=1
  Selector2 : Selector  InputPortWidth=3  IndexOptions=Index vector (dialog)  Indices=[2]  OutputSizes=1
  Selector3 : Selector  InputPortWidth=3  IndexOptions=Index vector (dialog)  Indices=[2]  OutputSizes=1
  Selector4 : Selector  InputPortWidth=9  IndexOptions=Index vector (dialog)  Indices=[6]  OutputSizes=1
  Selector5 : Selector  InputPortWidth=9  IndexOptions=Index vector (dialog)  Indices=[2 5 8]  OutputSizes=1
  Selector6 : Selector  InputPortWidth=9  IndexOptions=Index vector (dialog)  Indices=[3 6 9]  OutputSizes=1
  Sum : Sum  Inputs=|+-
  Sum1 : Sum  Inputs=|+-
  V : Scope
      settings: YMin=-3.5  YMax=7.5  SaveName=ScopeData3
  acc : Scope
      settings: YMin=-3.5  YMax=7.5  SaveName=ScopeData6
  Pos : Outport
  Vel : Outport  Port=2
  Acc : Outport  Port=3
  wires:
  Selector6/1 -> Acc/1
  Selector4/1 -> Mux1/2
  Selector3/1 -> Mux1/1
  Integrator1/1 -> Sum1/2
  Gain1/1 -> Selector3/1, Integrator1/1
  Sum1/1 -> Gain1/1
  Kalman Filter/2 -> Selector6/1, Selector5/1, Selector4/1
  In1/1 -> Sum/1, Kalman Filter/1
  Integrator/1 -> Sum/2, Pos/1
  Gain/1 -> Sum1/1, Integrator/1, Selector1/1
  Sum/1 -> Gain/1
  Mux/1 -> V/1
  Selector5/1 -> Vel/1, Selector2/1
  Mux1/1 -> acc/1
  Selector1/1 -> Mux/1
  Selector2/1 -> Mux/2
